simulink model "SystemComposerModel"  (R2022b)
settings: Solver=VariableStepAuto  StartTime=0.0  StopTime=10.0  RelTol=1e-3
(part 3 of 3)

== system SystemComposerModel/Competition/Trials/Prueba 5: Random obstacles/Trial Obstacles1 ==
  Bus Element In1 : Inport  PortName=Obstacles
  Doors : Subsystem  Description=They must be overcome by passing through the middle. The doors will be 1x1 meter square and elevated with the lower base half a meter off the ground.
      settings: PortSchema="{\"entries\":[{\"content\":{\"headerSize\":26,\"margin\":15,\"minimumSpacing\":25,\"sides\":[{\"content\":{\"connectorIds\":[]},\"type\":\"ConnectorPlacement.EquallySpacedRectSide\",\"uuid\":\"9053b2a7-4775-4bcf-9fc6-a069826350a9\"},{\"content\":{\"connectorIds\":[],\"side\":\"RIGHT\"},\"type\":\"ConnectorPlacement.EquallySpacedRectSide\",\"uuid\":\"b0969818-a4d3-4cbe-99b6-1949e99be80f\"},{\"content\":{\"connectorIds\":[],\"side\":\"TOP\"},\"type\":\"ConnectorPlacement.EquallySpacedRectSide\",\"uuid\":\"6c494ee9-6eb7-4ac7-893f-bc2d7701a0da\"}]},\"type\":\"ConnectorPlacement.EquallySpacedConnector\",\"uuid\":\"7a7eacf3-349d-4601-bac9-f57d73c6d0e2\"}],\"packageUris\":[\"http://schema.mathworks.com/mf0/Connector/R2020b\"],\"version\":\"1.0\"}"
  Split rectangle : Subsystem  Description=They can be red or blue. If they are red, you pass over them and if they are blue, you pass under them. The whole surface of the obstacle will be the same color and each rectangle will be 2x1m.
      settings: PortSchema="{\"entries\":[{\"content\":{\"headerSize\":26,\"margin\":15,\"minimumSpacing\":25,\"sides\":[{\"content\":{\"connectorIds\":[]},\"type\":\"ConnectorPlacement.EquallySpacedRectSide\",\"uuid\":\"9053b2a7-4775-4bcf-9fc6-a069826350a9\"},{\"content\":{\"connectorIds\":[],\"side\":\"RIGHT\"},\"type\":\"ConnectorPlacement.EquallySpacedRectSide\",\"uuid\":\"b0969818-a4d3-4cbe-99b6-1949e99be80f\"},{\"content\":{\"connectorIds\":[],\"side\":\"TOP\"},\"type\":\"ConnectorPlacement.EquallySpacedRectSide\",\"uuid\":\"6c494ee9-6eb7-4ac7-893f-bc2d7701a0da\"}]},\"type\":\"ConnectorPlacement.EquallySpacedConnector\",\"uuid\":\"7a7eacf3-349d-4601-bac9-f57d73c6d0e2\"}],\"packageUris\":[\"http://schema.mathworks.com/mf0/Connector/R2020b\"],\"version\":\"1.0\"}"
  Sticks : Subsystem  Description=They can be red or blue. If they are red they are passed on the left and if they are blue on the right. The stick will be 1.5 meters long and 4 cm wide. For a correct overcoming of the obstacle, the drone must not move more than 0.5 meters away from the sides and cannot exceed the height of the stick.
      settings: PortSchema="{\"entries\":[{\"content\":{\"headerSize\":26,\"margin\":15,\"minimumSpacing\":25,\"sides\":[{\"content\":{\"connectorIds\":[]},\"type\":\"ConnectorPlacement.EquallySpacedRectSide\",\"uuid\":\"9053b2a7-4775-4bcf-9fc6-a069826350a9\"},{\"content\":{\"connectorIds\":[],\"side\":\"RIGHT\"},\"type\":\"ConnectorPlacement.EquallySpacedRectSide\",\"uuid\":\"b0969818-a4d3-4cbe-99b6-1949e99be80f\"},{\"content\":{\"connectorIds\":[],\"side\":\"TOP\"},\"type\":\"ConnectorPlacement.EquallySpacedRectSide\",\"uuid\":\"6c494ee9-6eb7-4ac7-893f-bc2d7701a0da\"}]},\"type\":\"ConnectorPlacement.EquallySpacedConnector\",\"uuid\":\"7a7eacf3-349d-4601-bac9-f57d73c6d0e2\"}],\"packageUris\":[\"http://schema.mathworks.com/mf0/Connector/R2020b\"],\"version\":\"1.0\"}"

== system SystemComposerModel/Competition/Trials/Prueba 6: Freestyle/Rules ==

== system SystemComposerModel/Competition/Trials/Prueba 4: Predefined Obstacles/Trial Obstacles/Doors ==

== system SystemComposerModel/Competition/Trials/Prueba 4: Predefined Obstacles/Trial Obstacles/Split rectangle ==

== system SystemComposerModel/Competition/Trials/Prueba 4: Predefined Obstacles/Trial Obstacles/Sticks ==

== system SystemComposerModel/Competition/Trials/Prueba 5: Random obstacles/Trial Obstacles1/Doors ==

== system SystemComposerModel/Competition/Trials/Prueba 5: Random obstacles/Trial Obstacles1/Split rectangle ==

== system SystemComposerModel/Competition/Trials/Prueba 5: Random obstacles/Trial Obstacles1/Sticks ==
